simulink model "robot"  (Simulink 8.2)
settings: Solver=ode45  StartTime=0.0  StopTime=10  MaxStep=1e-3  RelTol=1e-3
settings Model: Creator=Jin  LastModifiedBy=Jin
settings DataIOCC: SignalLoggingSaveFormat=Dataset
settings OptimizationCC: ExpressionDepthLimit=128
settings DebuggingCC: FcnCallInpInsideContextMsg=EnableAllAsError  StateNameClashWarn=none
settings GRTTargetCC: CombineOutputUpdateFcns=on  GRTInterface=off

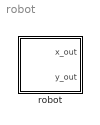
== system robot ==
  robot : Stateflow chart  TreatAsAtomicUnit=on

== stateflow chart robot ==
  settings: updateMethod=CONTINUOUS
  state Move
    du:
    x_dot = 5 * sin(theta);
    y_dot = 5 * cos(theta);
    theta_dot  = 0.9;
    x_out = x;
    y_out = y;
  state Stop
    du:
    x_dot = 0;
    y_dot = 0;
    theta_dot = 0;
    x_out = x;
    y_out = y;
  (default) -> Move : {theta = 0;
      | x = 0;
      | y= 0;}
  Move -> Stop : [y >= 12 *x *x - 54* x + 65]
  data: x local double; y local double; theta local double; x_out output double; y_out output double
  data x settings: updateMethod=SF_CONTINUOUS_TIME_DATA
  data y settings: updateMethod=SF_CONTINUOUS_TIME_DATA
  data theta settings: updateMethod=SF_CONTINUOUS_TIME_DATA
